simulink model "TST_AirHt_Ctl"  (R2016b)
settings: Solver=FixedStepDiscrete  StartTime=0.0  StopTime=simTime  FixedStep=sampleTime  RelTol=1e-3
values from neighbouring files (symbols this model uses):
  testCase = 1    [initTST_AirHt_Ctl_001.m]    (also in initTST_AirHt_Ctl_002.m = 2; initTST_AirHt_Ctl_003.m = 3; initTST_AirHt_Ctl_004.m = 4; initTST_AirHt_Ctl_005.m = 5)
libraries: simulink x53, UnitTest_Lib x26
(part 1 of 4)
settings Model: Creator=zhengjinyan  LastModifiedBy=zhengjinyan
settings DebuggingCC: SignalRangeChecking=error

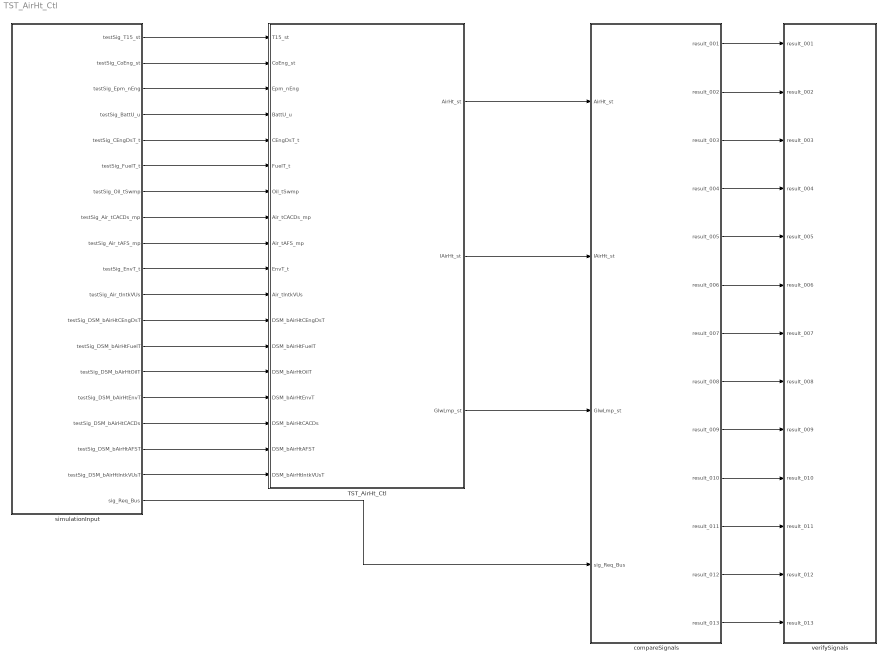
== system TST_AirHt_Ctl ==
  TST_AirHt_Ctl : Subsystem
  compareSignals : Subsystem
  simulationInput : Subsystem
  verifySignals : Subsystem
  wires:
  simulationInput/1(testSig_T15_st) -> TST_AirHt_Ctl/1(T15_st)
  simulationInput/2(testSig_CoEng_st) -> TST_AirHt_Ctl/2(CoEng_st)
  simulationInput/3(testSig_Epm_nEng) -> TST_AirHt_Ctl/3(Epm_nEng)
  simulationInput/4(testSig_BattU_u) -> TST_AirHt_Ctl/4(BattU_u)
  simulationInput/5(testSig_CEngDsT_t) -> TST_AirHt_Ctl/5(CEngDsT_t)
  simulationInput/6(testSig_FuelT_t) -> TST_AirHt_Ctl/6(FuelT_t)
  simulationInput/7(testSig_Oil_tSwmp) -> TST_AirHt_Ctl/7(Oil_tSwmp)
  simulationInput/8(testSig_Air_tCACDs_mp) -> TST_AirHt_Ctl/8(Air_tCACDs_mp)
  simulationInput/9(testSig_Air_tAFS_mp) -> TST_AirHt_Ctl/9(Air_tAFS_mp)
  simulationInput/10(testSig_EnvT_t) -> TST_AirHt_Ctl/10(EnvT_t)
  simulationInput/11(testSig_Air_tIntkVUs) -> TST_AirHt_Ctl/11(Air_tIntkVUs)
  simulationInput/12(testSig_DSM_bAirHtCEngDsT) -> TST_AirHt_Ctl/12(DSM_bAirHtCEngDsT)
  simulationInput/13(testSig_DSM_bAirHtFuelT) -> TST_AirHt_Ctl/13(DSM_bAirHtFuelT)
  simulationInput/14(testSig_DSM_bAirHtOilT) -> TST_AirHt_Ctl/14(DSM_bAirHtOilT)
  simulationInput/15(testSig_DSM_bAirHtEnvT) -> TST_AirHt_Ctl/15(DSM_bAirHtEnvT)
  simulationInput/16(testSig_DSM_bAirHtCACDs) -> TST_AirHt_Ctl/16(DSM_bAirHtCACDs)
  simulationInput/17(testSig_DSM_bAirHtAFST) -> TST_AirHt_Ctl/17(DSM_bAirHtAFST)
  simulationInput/18(testSig_DSM_bAirHtIntkVUsT) -> TST_AirHt_Ctl/18(DSM_bAirHtIntkVUsT)
  TST_AirHt_Ctl/1(AirHt_st) -> compareSignals/1(AirHt_st)
  TST_AirHt_Ctl/2(IAirHt_st) -> compareSignals/2(IAirHt_st)
  TST_AirHt_Ctl/3(GlwLmp_st) -> compareSignals/3(GlwLmp_st)
  simulationInput/19(sig_Req_Bus) -> compareSignals/4(sig_Req_Bus)
  compareSignals/1(result_001) -> verifySignals/1(result_001)
  compareSignals/2(result_002) -> verifySignals/2(result_002)
  compareSignals/3(result_003) -> verifySignals/3(result_003)
  compareSignals/4(result_004) -> verifySignals/4(result_004)
  compareSignals/5(result_005) -> verifySignals/5(result_005)
  compareSignals/6(result_006) -> verifySignals/6(result_006)
  compareSignals/7(result_007) -> verifySignals/7(result_007)
  compareSignals/8(result_008) -> verifySignals/8(result_008)
  compareSignals/9(result_009) -> verifySignals/9(result_009)
  compareSignals/10(result_010) -> verifySignals/10(result_010)
  compareSignals/11(result_011) -> verifySignals/11(result_011)
  compareSignals/12(result_012) -> verifySignals/12(result_012)
  compareSignals/13(result_013) -> verifySignals/13(result_013)

== system TST_AirHt_Ctl/TST_AirHt_Ctl ==
  T15_st : Inport
  CoEng_st : Inport  Port=2
  Epm_nEng : Inport  Port=3
  BattU_u : Inport  Port=4
  CEngDsT_t : Inport  Port=5
  FuelT_t : Inport  Port=6
  Oil_tSwmp : Inport  Port=7
  Air_tCACDs_mp : Inport  Port=8
  Air_tAFS_mp : Inport  Port=9
  EnvT_t : Inport  Port=10
  Air_tIntkVUs : Inport  Port=11
  DSM_bAirHtCEngDsT : Inport  Port=12
  DSM_bAirHtFuelT : Inport  Port=13
  DSM_bAirHtOilT : Inport  Port=14
  DSM_bAirHtEnvT : Inport  Port=15
  DSM_bAirHtCACDs : Inport  Port=16
  DSM_bAirHtAFST : Inport  Port=17
  DSM_bAirHtIntkVUsT : Inport  Port=18
  AirHt_Ctl : ModelReference  ModelNameDialog=AirHt_Ctl  SimulationMode=Normal  ModelReferenceVersion=1.145  TriggerPortName=function  TriggerPortTriggerType=function-call  TriggerPortStatesWhenEnabling=held
  Function_Call : simulink/Ports & Subsystems/Function-Call Generator  sample_time=sampleTime  numberOfIterations=1
  AirHt_st : Outport
  IAirHt_st : Outport  Port=2
  GlwLmp_st : Outport  Port=3
  wires:
  Function_Call/1 -> AirHt_Ctl/Trigger
  T15_st/1 -> AirHt_Ctl/1
  CoEng_st/1 -> AirHt_Ctl/2
  Epm_nEng/1 -> AirHt_Ctl/3
  BattU_u/1 -> AirHt_Ctl/4
  CEngDsT_t/1 -> AirHt_Ctl/5
  FuelT_t/1 -> AirHt_Ctl/6
  Oil_tSwmp/1 -> AirHt_Ctl/7
  Air_tCACDs_mp/1 -> AirHt_Ctl/8
  Air_tAFS_mp/1 -> AirHt_Ctl/9
  EnvT_t/1 -> AirHt_Ctl/10
  Air_tIntkVUs/1 -> AirHt_Ctl/11
  DSM_bAirHtCEngDsT/1 -> AirHt_Ctl/12
  DSM_bAirHtFuelT/1 -> AirHt_Ctl/13
  DSM_bAirHtOilT/1 -> AirHt_Ctl/14
  DSM_bAirHtEnvT/1 -> AirHt_Ctl/15
  DSM_bAirHtCACDs/1 -> AirHt_Ctl/16
  DSM_bAirHtAFST/1 -> AirHt_Ctl/17
  DSM_bAirHtIntkVUsT/1 -> AirHt_Ctl/18
  AirHt_Ctl/1 -> AirHt_st/1
  AirHt_Ctl/2 -> IAirHt_st/1
  AirHt_Ctl/3 -> GlwLmp_st/1

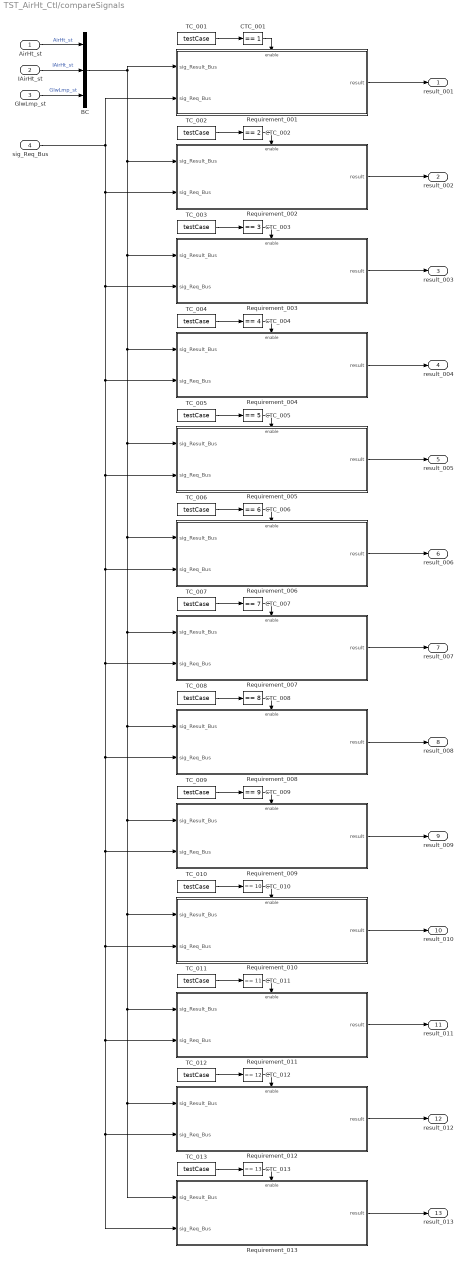
== system TST_AirHt_Ctl/compareSignals ==
  AirHt_st : Inport
  IAirHt_st : Inport  Port=2
  GlwLmp_st : Inport  Port=3
  sig_Req_Bus : Inport  Port=4
  BC : BusCreator  Inputs=3
  CTC_001 : simulink/Logic and Bit Operations/Compare To Constant  relop===  const=1  OutDataTypeStr=boolean
  CTC_002 : simulink/Logic and Bit Operations/Compare To Constant  relop===  const=2  OutDataTypeStr=boolean
  CTC_003 : simulink/Logic and Bit Operations/Compare To Constant  relop===  const=3  OutDataTypeStr=boolean
  CTC_004 : simulink/Logic and Bit Operations/Compare To Constant  relop===  const=4  OutDataTypeStr=boolean
  CTC_005 : simulink/Logic and Bit Operations/Compare To Constant  relop===  const=5  OutDataTypeStr=boolean
  CTC_006 : simulink/Logic and Bit Operations/Compare To Constant  relop===  const=6  OutDataTypeStr=boolean
  CTC_007 : simulink/Logic and Bit Operations/Compare To Constant  relop===  const=7  OutDataTypeStr=boolean
  CTC_008 : simulink/Logic and Bit Operations/Compare To Constant  relop===  const=8  OutDataTypeStr=boolean
  CTC_009 : simulink/Logic and Bit Operations/Compare To Constant  relop===  const=9  OutDataTypeStr=boolean
  CTC_010 : simulink/Logic and Bit Operations/Compare To Constant  relop===  const=10  OutDataTypeStr=boolean
  CTC_011 : simulink/Logic and Bit Operations/Compare To Constant  relop===  const=11  OutDataTypeStr=boolean
  CTC_012 : simulink/Logic and Bit Operations/Compare To Constant  relop===  const=12  OutDataTypeStr=boolean
  CTC_013 : simulink/Logic and Bit Operations/Compare To Constant  relop===  const=13  OutDataTypeStr=boolean
  Requirement_001 : Subsystem
  Requirement_002 : Subsystem
  Requirement_003 : Subsystem
  Requirement_004 : Subsystem
  Requirement_005 : Subsystem
  Requirement_006 : Subsystem
  Requirement_007 : Subsystem
  Requirement_008 : Subsystem
  Requirement_009 : Subsystem
  Requirement_010 : Subsystem
  Requirement_011 : Subsystem
  Requirement_012 : Subsystem
  Requirement_013 : Subsystem
  TC_001 : Constant  Value=testCase
  TC_002 : Constant  Value=testCase
  TC_003 : Constant  Value=testCase
  TC_004 : Constant  Value=testCase
  TC_005 : Constant  Value=testCase
  TC_006 : Constant  Value=testCase
  TC_007 : Constant  Value=testCase
  TC_008 : Constant  Value=testCase
  TC_009 : Constant  Value=testCase
  TC_010 : Constant  Value=testCase
  TC_011 : Constant  Value=testCase
  TC_012 : Constant  Value=testCase
  TC_013 : Constant  Value=testCase
  result_001 : Outport
  result_002 : Outport  Port=2
  result_003 : Outport  Port=3
  result_004 : Outport  Port=4
  result_005 : Outport  Port=5
  result_006 : Outport  Port=6
  result_007 : Outport  Port=7
  result_008 : Outport  Port=8
  result_009 : Outport  Port=9
  result_010 : Outport  Port=10
  result_011 : Outport  Port=11
  result_012 : Outport  Port=12
  result_013 : Outport  Port=13
  wires:
  AirHt_st/1 -> BC/1  "AirHt_st"
  IAirHt_st/1 -> BC/2  "IAirHt_st"
  GlwLmp_st/1 -> BC/3  "GlwLmp_st"
  TC_001/1 -> CTC_001/1
  CTC_001/1 -> Requirement_001/Enable
  sig_Req_Bus/1 -> Requirement_012/2(sig_Req_Bus), Requirement_013/2(sig_Req_Bus), Requirement_011/2(sig_Req_Bus), Requirement_010/2(sig_Req_Bus), Requirement_009/2(sig_Req_Bus), Requirement_008/2(sig_Req_Bus), Requirement_007/2(sig_Req_Bus), Requirement_006/2(sig_Req_Bus), Requirement_005/2(sig_Req_Bus), Requirement_004/2(sig_Req_Bus), Requirement_003/2(sig_Req_Bus), Requirement_002/2(sig_Req_Bus), Requirement_001/2(sig_Req_Bus)
  BC/1 -> Requirement_012/1(sig_Result_Bus), Requirement_013/1(sig_Result_Bus), Requirement_011/1(sig_Result_Bus), Requirement_010/1(sig_Result_Bus), Requirement_009/1(sig_Result_Bus), Requirement_008/1(sig_Result_Bus), Requirement_007/1(sig_Result_Bus), Requirement_006/1(sig_Result_Bus), Requirement_005/1(sig_Result_Bus), Requirement_004/1(sig_Result_Bus), Requirement_003/1(sig_Result_Bus), Requirement_002/1(sig_Result_Bus), Requirement_001/1(sig_Result_Bus)
  Requirement_001/1(result) -> result_001/1
  TC_002/1 -> CTC_002/1
  CTC_002/1 -> Requirement_002/Enable
  Requirement_002/1(result) -> result_002/1
  TC_003/1 -> CTC_003/1
  CTC_003/1 -> Requirement_003/Enable
  Requirement_003/1(result) -> result_003/1
  TC_004/1 -> CTC_004/1
  CTC_004/1 -> Requirement_004/Enable
  Requirement_004/1(result) -> result_004/1
  TC_005/1 -> CTC_005/1
  CTC_005/1 -> Requirement_005/Enable
  Requirement_005/1(result) -> result_005/1
  TC_006/1 -> CTC_006/1
  CTC_006/1 -> Requirement_006/Enable
  Requirement_006/1(result) -> result_006/1
  TC_007/1 -> CTC_007/1
  CTC_007/1 -> Requirement_007/Enable
  Requirement_007/1(result) -> result_007/1
  TC_008/1 -> CTC_008/1
  CTC_008/1 -> Requirement_008/Enable
  Requirement_008/1(result) -> result_008/1
  TC_009/1 -> CTC_009/1
  CTC_009/1 -> Requirement_009/Enable
  Requirement_009/1(result) -> result_009/1
  TC_010/1 -> CTC_010/1
  CTC_010/1 -> Requirement_010/Enable
  Requirement_010/1(result) -> result_010/1
  TC_011/1 -> CTC_011/1
  CTC_011/1 -> Requirement_011/Enable
  Requirement_011/1(result) -> result_011/1
  TC_012/1 -> CTC_012/1
  CTC_012/1 -> Requirement_012/Enable
  Requirement_012/1(result) -> result_012/1
  TC_013/1 -> CTC_013/1
  CTC_013/1 -> Requirement_013/Enable
  Requirement_013/1(result) -> result_013/1

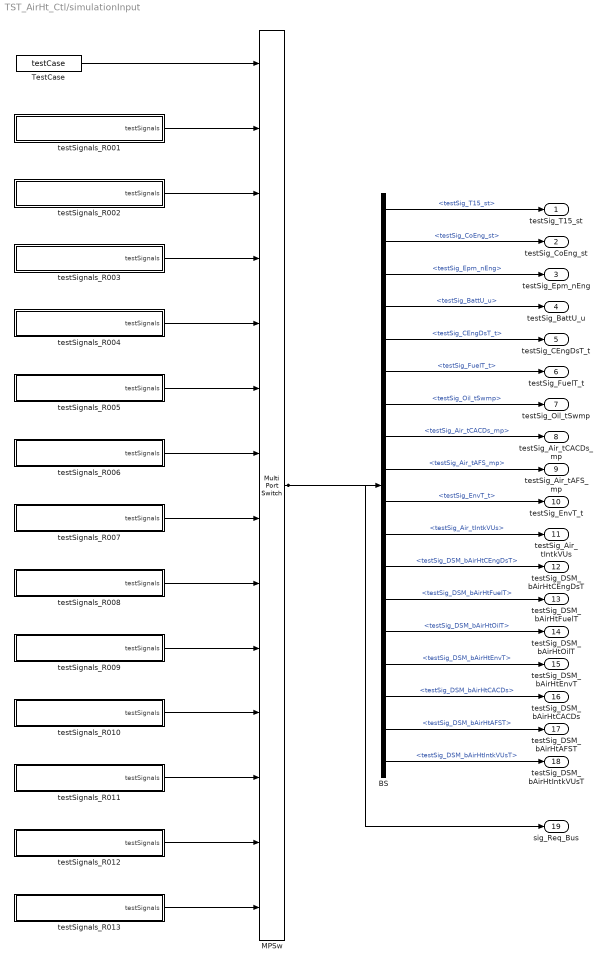
== system TST_AirHt_Ctl/simulationInput ==
  BS : BusSelector  OutputSignals=testSig_T15_st,testSig_CoEng_st,testSig_Epm_nEng,testSig_BattU_u,testSig_CEngDsT_t,testSig_FuelT_t,testSig_Oil_tSwmp,testSig_Air_tCACDs_mp,testSig_Air_tAFS_mp,testSig_EnvT_t,testSig_Air_tIntkVUs,testSig_DSM_bAirHtCEngDsT,testSig_DSM_bAirHtFuelT,testSig_DSM_bAirHtOilT,testSig_DSM_bAirHtEnvT,testSig_DSM_bAirHtCACDs,testSig_DSM_bAirHtAFST,testSig_DSM_bAirHtIntkVUsT
  MPSw : MultiPortSwitch  Inputs=13  SaturateOnIntegerOverflow=on  InputSameDT=on
  TestCase : Constant  Value=testCase
  testSignals_R001 : Subsystem
  testSignals_R002 : Subsystem
  testSignals_R003 : Subsystem
  testSignals_R004 : Subsystem
  testSignals_R005 : Subsystem
  testSignals_R006 : Subsystem
  testSignals_R007 : Subsystem
  testSignals_R008 : Subsystem
  testSignals_R009 : Subsystem
  testSignals_R010 : Subsystem
  testSignals_R011 : Subsystem
  testSignals_R012 : Subsystem
  testSignals_R013 : Subsystem
  testSig_T15_st : Outport
  testSig_CoEng_st : Outport  Port=2
  testSig_Epm_nEng : Outport  Port=3
  testSig_BattU_u : Outport  Port=4
  testSig_CEngDsT_t : Outport  Port=5
  testSig_FuelT_t : Outport  Port=6
  testSig_Oil_tSwmp : Outport  Port=7
  testSig_Air_tCACDs_mp : Outport  Port=8
  testSig_Air_tAFS_mp : Outport  Port=9
  testSig_EnvT_t : Outport  Port=10
  testSig_Air_tIntkVUs : Outport  Port=11
  testSig_DSM_bAirHtCEngDsT : Outport  Port=12
  testSig_DSM_bAirHtFuelT : Outport  Port=13
  testSig_DSM_bAirHtOilT : Outport  Port=14
  testSig_DSM_bAirHtEnvT : Outport  Port=15
  testSig_DSM_bAirHtCACDs : Outport  Port=16
  testSig_DSM_bAirHtAFST : Outport  Port=17
  testSig_DSM_bAirHtIntkVUsT : Outport  Port=18
  sig_Req_Bus : Outport  Port=19
  wires:
  BS/1 -> testSig_T15_st/1  "<testSig_T15_st>"
  BS/2 -> testSig_CoEng_st/1  "<testSig_CoEng_st>"
  BS/3 -> testSig_Epm_nEng/1  "<testSig_Epm_nEng>"
  BS/4 -> testSig_BattU_u/1  "<testSig_BattU_u>"
  BS/5 -> testSig_CEngDsT_t/1  "<testSig_CEngDsT_t>"
  BS/6 -> testSig_FuelT_t/1  "<testSig_FuelT_t>"
  BS/7 -> testSig_Oil_tSwmp/1  "<testSig_Oil_tSwmp>"
  BS/8 -> testSig_Air_tCACDs_mp/1  "<testSig_Air_tCACDs_mp>"
  BS/9 -> testSig_Air_tAFS_mp/1  "<testSig_Air_tAFS_mp>"
  BS/10 -> testSig_EnvT_t/1  "<testSig_EnvT_t>"
  BS/11 -> testSig_Air_tIntkVUs/1  "<testSig_Air_tIntkVUs>"
  BS/12 -> testSig_DSM_bAirHtCEngDsT/1  "<testSig_DSM_bAirHtCEngDsT>"
  BS/13 -> testSig_DSM_bAirHtFuelT/1  "<testSig_DSM_bAirHtFuelT>"
  BS/14 -> testSig_DSM_bAirHtOilT/1  "<testSig_DSM_bAirHtOilT>"
  BS/15 -> testSig_DSM_bAirHtEnvT/1  "<testSig_DSM_bAirHtEnvT>"
  BS/16 -> testSig_DSM_bAirHtCACDs/1  "<testSig_DSM_bAirHtCACDs>"
  BS/17 -> testSig_DSM_bAirHtAFST/1  "<testSig_DSM_bAirHtAFST>"
  BS/18 -> testSig_DSM_bAirHtIntkVUsT/1  "<testSig_DSM_bAirHtIntkVUsT>"
  MPSw/1 -> BS/1, sig_Req_Bus/1
  TestCase/1 -> MPSw/1
  testSignals_R001/1(testSignals) -> MPSw/2
  testSignals_R002/1(testSignals) -> MPSw/3
  testSignals_R003/1(testSignals) -> MPSw/4
  testSignals_R004/1(testSignals) -> MPSw/5
  testSignals_R005/1(testSignals) -> MPSw/6
  testSignals_R006/1(testSignals) -> MPSw/7
  testSignals_R007/1(testSignals) -> MPSw/8
  testSignals_R008/1(testSignals) -> MPSw/9
  testSignals_R009/1(testSignals) -> MPSw/10
  testSignals_R010/1(testSignals) -> MPSw/11
  testSignals_R011/1(testSignals) -> MPSw/12
  testSignals_R012/1(testSignals) -> MPSw/13
  testSignals_R013/1(testSignals) -> MPSw/14

== system TST_AirHt_Ctl/verifySignals ==
  result_001 : Inport
  result_002 : Inport  Port=2
  result_003 : Inport  Port=3
  result_004 : Inport  Port=4
  result_005 : Inport  Port=5
  result_006 : Inport  Port=6
  result_007 : Inport  Port=7
  result_008 : Inport  Port=8
  result_009 : Inport  Port=9
  result_010 : Inport  Port=10
  result_011 : Inport  Port=11
  result_012 : Inport  Port=12
  result_013 : Inport  Port=13
  Assertion_001 : Assertion  Enabled=off
  Assertion_002 : Assertion  Enabled=off
  Assertion_003 : Assertion  Enabled=off
  Assertion_004 : Assertion  Enabled=off
  Assertion_005 : Assertion  Enabled=off
  Assertion_006 : Assertion  Enabled=off
  Assertion_007 : Assertion  Enabled=off
  Assertion_008 : Assertion  Enabled=off
  Assertion_009 : Assertion  Enabled=off
  Assertion_010 : Assertion  Enabled=off
  Assertion_011 : Assertion  Enabled=off
  Assertion_012 : Assertion  Enabled=off
  Assertion_013 : Assertion  Enabled=off
  wires:
  result_001/1 -> Assertion_001/1
  result_002/1 -> Assertion_002/1
  result_003/1 -> Assertion_003/1
  result_004/1 -> Assertion_004/1
  result_005/1 -> Assertion_005/1
  result_006/1 -> Assertion_006/1
  result_007/1 -> Assertion_007/1
  result_008/1 -> Assertion_008/1
  result_009/1 -> Assertion_009/1
  result_010/1 -> Assertion_010/1
  result_011/1 -> Assertion_011/1
  result_012/1 -> Assertion_012/1
  result_013/1 -> Assertion_013/1

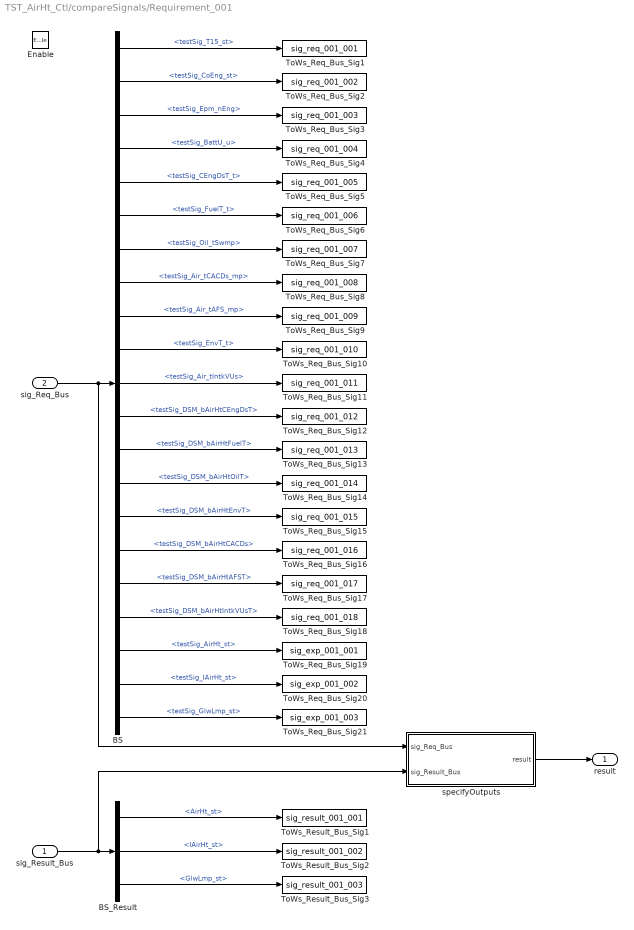
== system TST_AirHt_Ctl/compareSignals/Requirement_001 ==
  sig_Result_Bus : Inport
  sig_Req_Bus : Inport  Port=2
  Enable : EnablePort
  BS : BusSelector  OutputSignals=testSig_T15_st,testSig_CoEng_st,testSig_Epm_nEng,testSig_BattU_u,testSig_CEngDsT_t,testSig_FuelT_t,testSig_Oil_tSwmp,testSig_Air_tCACDs_mp,testSig_Air_tAFS_mp,testSig_EnvT_t,testSig_Air_tIntkVUs,testSig_DSM_bAirHtCEngDsT,testSig_DSM_bAirHtFuelT,testSig_DSM_bAirHtOilT,testSig_DSM_bAirHtEnvT,testSig_DSM_bAirHtCACDs,testSig_DSM_bAirHtAFST,testSig_DSM_bAirHtIntkVUsT,testSig_AirHt_st,testSig_IAirHt_st,testSig_GlwLmp_st
  BS_Result : BusSelector  OutputSignals=AirHt_st,IAirHt_st,GlwLmp_st
  ToWs_Req_Bus_Sig1 : ToWorkspace  VariableName=sig_req_001_001  SaveFormat=Structure With Time
  ToWs_Req_Bus_Sig10 : ToWorkspace  VariableName=sig_req_001_010  SaveFormat=Structure With Time
  ToWs_Req_Bus_Sig11 : ToWorkspace  VariableName=sig_req_001_011  SaveFormat=Structure With Time
  ToWs_Req_Bus_Sig12 : ToWorkspace  VariableName=sig_req_001_012  SaveFormat=Structure With Time
  ToWs_Req_Bus_Sig13 : ToWorkspace  VariableName=sig_req_001_013  SaveFormat=Structure With Time
  ToWs_Req_Bus_Sig14 : ToWorkspace  VariableName=sig_req_001_014  SaveFormat=Structure With Time
  ToWs_Req_Bus_Sig15 : ToWorkspace  VariableName=sig_req_001_015  SaveFormat=Structure With Time
  ToWs_Req_Bus_Sig16 : ToWorkspace  VariableName=sig_req_001_016  SaveFormat=Structure With Time
  ToWs_Req_Bus_Sig17 : ToWorkspace  VariableName=sig_req_001_017  SaveFormat=Structure With Time
  ToWs_Req_Bus_Sig18 : ToWorkspace  VariableName=sig_req_001_018  SaveFormat=Structure With Time
  ToWs_Req_Bus_Sig19 : ToWorkspace  VariableName=sig_exp_001_001  SaveFormat=Structure With Time
  ToWs_Req_Bus_Sig2 : ToWorkspace  VariableName=sig_req_001_002  SaveFormat=Structure With Time
  ToWs_Req_Bus_Sig20 : ToWorkspace  VariableName=sig_exp_001_002  SaveFormat=Structure With Time
  ToWs_Req_Bus_Sig21 : ToWorkspace  VariableName=sig_exp_001_003  SaveFormat=Structure With Time
  ToWs_Req_Bus_Sig3 : ToWorkspace  VariableName=sig_req_001_003  SaveFormat=Structure With Time
  ToWs_Req_Bus_Sig4 : ToWorkspace  VariableName=sig_req_001_004  SaveFormat=Structure With Time
  ToWs_Req_Bus_Sig5 : ToWorkspace  VariableName=sig_req_001_005  SaveFormat=Structure With Time
  ToWs_Req_Bus_Sig6 : ToWorkspace  VariableName=sig_req_001_006  SaveFormat=Structure With Time
  ToWs_Req_Bus_Sig7 : ToWorkspace  VariableName=sig_req_001_007  SaveFormat=Structure With Time
  ToWs_Req_Bus_Sig8 : ToWorkspace  VariableName=sig_req_001_008  SaveFormat=Structure With Time
  ToWs_Req_Bus_Sig9 : ToWorkspace  VariableName=sig_req_001_009  SaveFormat=Structure With Time
  ToWs_Result_Bus_Sig1 : ToWorkspace  VariableName=sig_result_001_001  SaveFormat=Structure With Time
  ToWs_Result_Bus_Sig2 : ToWorkspace  VariableName=sig_result_001_002  SaveFormat=Structure With Time
  ToWs_Result_Bus_Sig3 : ToWorkspace  VariableName=sig_result_001_003  SaveFormat=Structure With Time
  specifyOutputs : Subsystem
  result : Outport
  wires:
  sig_Req_Bus/1 -> BS/1, specifyOutputs/1(sig_Req_Bus)
  BS/1 -> ToWs_Req_Bus_Sig1/1  "<testSig_T15_st>"
  BS/2 -> ToWs_Req_Bus_Sig2/1  "<testSig_CoEng_st>"
  BS/3 -> ToWs_Req_Bus_Sig3/1  "<testSig_Epm_nEng>"
  BS/4 -> ToWs_Req_Bus_Sig4/1  "<testSig_BattU_u>"
  BS/5 -> ToWs_Req_Bus_Sig5/1  "<testSig_CEngDsT_t>"
  BS/6 -> ToWs_Req_Bus_Sig6/1  "<testSig_FuelT_t>"
  BS/7 -> ToWs_Req_Bus_Sig7/1  "<testSig_Oil_tSwmp>"
  BS/8 -> ToWs_Req_Bus_Sig8/1  "<testSig_Air_tCACDs_mp>"
  BS/9 -> ToWs_Req_Bus_Sig9/1  "<testSig_Air_tAFS_mp>"
  BS/10 -> ToWs_Req_Bus_Sig10/1  "<testSig_EnvT_t>"
  BS/11 -> ToWs_Req_Bus_Sig11/1  "<testSig_Air_tIntkVUs>"
  BS/12 -> ToWs_Req_Bus_Sig12/1  "<testSig_DSM_bAirHtCEngDsT>"
  BS/13 -> ToWs_Req_Bus_Sig13/1  "<testSig_DSM_bAirHtFuelT>"
  BS/14 -> ToWs_Req_Bus_Sig14/1  "<testSig_DSM_bAirHtOilT>"
  BS/15 -> ToWs_Req_Bus_Sig15/1  "<testSig_DSM_bAirHtEnvT>"
  BS/16 -> ToWs_Req_Bus_Sig16/1  "<testSig_DSM_bAirHtCACDs>"
  BS/17 -> ToWs_Req_Bus_Sig17/1  "<testSig_DSM_bAirHtAFST>"
  BS/18 -> ToWs_Req_Bus_Sig18/1  "<testSig_DSM_bAirHtIntkVUsT>"
  BS/19 -> ToWs_Req_Bus_Sig19/1  "<testSig_AirHt_st>"
  BS/20 -> ToWs_Req_Bus_Sig20/1  "<testSig_IAirHt_st>"
  BS/21 -> ToWs_Req_Bus_Sig21/1  "<testSig_GlwLmp_st>"
  sig_Result_Bus/1 -> BS_Result/1, specifyOutputs/2(sig_Result_Bus)
  BS_Result/1 -> ToWs_Result_Bus_Sig1/1  "<AirHt_st>"
  BS_Result/2 -> ToWs_Result_Bus_Sig2/1  "<IAirHt_st>"
  BS_Result/3 -> ToWs_Result_Bus_Sig3/1  "<GlwLmp_st>"
  specifyOutputs/1(result) -> result/1

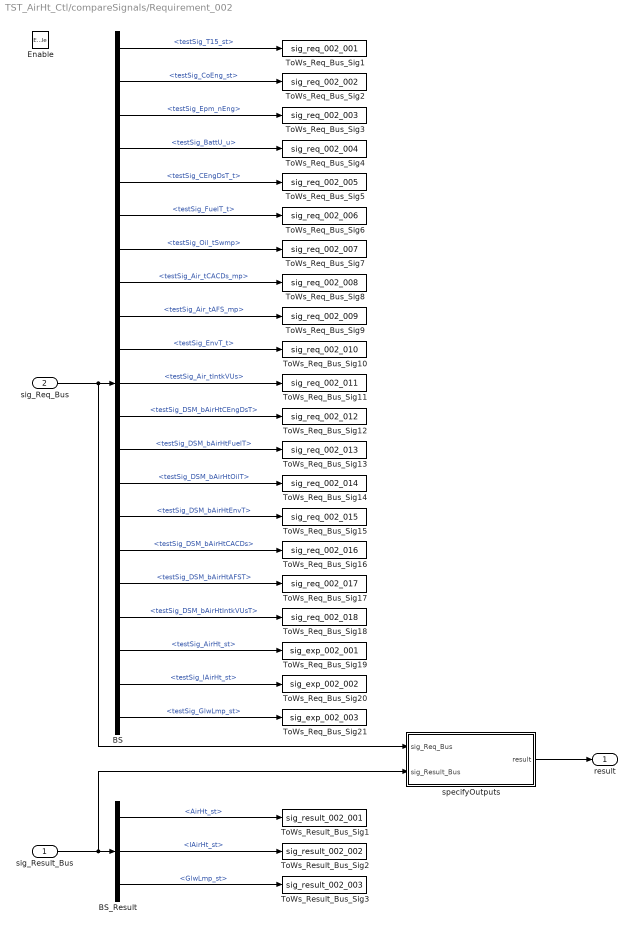
== system TST_AirHt_Ctl/compareSignals/Requirement_002 ==
  sig_Result_Bus : Inport
  sig_Req_Bus : Inport  Port=2
  Enable : EnablePort
  BS : BusSelector  OutputSignals=testSig_T15_st,testSig_CoEng_st,testSig_Epm_nEng,testSig_BattU_u,testSig_CEngDsT_t,testSig_FuelT_t,testSig_Oil_tSwmp,testSig_Air_tCACDs_mp,testSig_Air_tAFS_mp,testSig_EnvT_t,testSig_Air_tIntkVUs,testSig_DSM_bAirHtCEngDsT,testSig_DSM_bAirHtFuelT,testSig_DSM_bAirHtOilT,testSig_DSM_bAirHtEnvT,testSig_DSM_bAirHtCACDs,testSig_DSM_bAirHtAFST,testSig_DSM_bAirHtIntkVUsT,testSig_AirHt_st,testSig_IAirHt_st,testSig_GlwLmp_st
  BS_Result : BusSelector  OutputSignals=AirHt_st,IAirHt_st,GlwLmp_st
  ToWs_Req_Bus_Sig1 : ToWorkspace  VariableName=sig_req_002_001  SaveFormat=Structure With Time
  ToWs_Req_Bus_Sig10 : ToWorkspace  VariableName=sig_req_002_010  SaveFormat=Structure With Time
  ToWs_Req_Bus_Sig11 : ToWorkspace  VariableName=sig_req_002_011  SaveFormat=Structure With Time
  ToWs_Req_Bus_Sig12 : ToWorkspace  VariableName=sig_req_002_012  SaveFormat=Structure With Time
  ToWs_Req_Bus_Sig13 : ToWorkspace  VariableName=sig_req_002_013  SaveFormat=Structure With Time
  ToWs_Req_Bus_Sig14 : ToWorkspace  VariableName=sig_req_002_014  SaveFormat=Structure With Time
  ToWs_Req_Bus_Sig15 : ToWorkspace  VariableName=sig_req_002_015  SaveFormat=Structure With Time
  ToWs_Req_Bus_Sig16 : ToWorkspace  VariableName=sig_req_002_016  SaveFormat=Structure With Time
  ToWs_Req_Bus_Sig17 : ToWorkspace  VariableName=sig_req_002_017  SaveFormat=Structure With Time
  ToWs_Req_Bus_Sig18 : ToWorkspace  VariableName=sig_req_002_018  SaveFormat=Structure With Time
  ToWs_Req_Bus_Sig19 : ToWorkspace  VariableName=sig_exp_002_001  SaveFormat=Structure With Time
  ToWs_Req_Bus_Sig2 : ToWorkspace  VariableName=sig_req_002_002  SaveFormat=Structure With Time
  ToWs_Req_Bus_Sig20 : ToWorkspace  VariableName=sig_exp_002_002  SaveFormat=Structure With Time
  ToWs_Req_Bus_Sig21 : ToWorkspace  VariableName=sig_exp_002_003  SaveFormat=Structure With Time
  ToWs_Req_Bus_Sig3 : ToWorkspace  VariableName=sig_req_002_003  SaveFormat=Structure With Time
  ToWs_Req_Bus_Sig4 : ToWorkspace  VariableName=sig_req_002_004  SaveFormat=Structure With Time
  ToWs_Req_Bus_Sig5 : ToWorkspace  VariableName=sig_req_002_005  SaveFormat=Structure With Time
  ToWs_Req_Bus_Sig6 : ToWorkspace  VariableName=sig_req_002_006  SaveFormat=Structure With Time
  ToWs_Req_Bus_Sig7 : ToWorkspace  VariableName=sig_req_002_007  SaveFormat=Structure With Time
  ToWs_Req_Bus_Sig8 : ToWorkspace  VariableName=sig_req_002_008  SaveFormat=Structure With Time
  ToWs_Req_Bus_Sig9 : ToWorkspace  VariableName=sig_req_002_009  SaveFormat=Structure With Time
  ToWs_Result_Bus_Sig1 : ToWorkspace  VariableName=sig_result_002_001  SaveFormat=Structure With Time
  ToWs_Result_Bus_Sig2 : ToWorkspace  VariableName=sig_result_002_002  SaveFormat=Structure With Time
  ToWs_Result_Bus_Sig3 : ToWorkspace  VariableName=sig_result_002_003  SaveFormat=Structure With Time
  specifyOutputs : Subsystem
  result : Outport
  wires:
  sig_Req_Bus/1 -> BS/1, specifyOutputs/1(sig_Req_Bus)
  BS/1 -> ToWs_Req_Bus_Sig1/1  "<testSig_T15_st>"
  BS/2 -> ToWs_Req_Bus_Sig2/1  "<testSig_CoEng_st>"
  BS/3 -> ToWs_Req_Bus_Sig3/1  "<testSig_Epm_nEng>"
  BS/4 -> ToWs_Req_Bus_Sig4/1  "<testSig_BattU_u>"
  BS/5 -> ToWs_Req_Bus_Sig5/1  "<testSig_CEngDsT_t>"
  BS/6 -> ToWs_Req_Bus_Sig6/1  "<testSig_FuelT_t>"
  BS/7 -> ToWs_Req_Bus_Sig7/1  "<testSig_Oil_tSwmp>"
  BS/8 -> ToWs_Req_Bus_Sig8/1  "<testSig_Air_tCACDs_mp>"
  BS/9 -> ToWs_Req_Bus_Sig9/1  "<testSig_Air_tAFS_mp>"
  BS/10 -> ToWs_Req_Bus_Sig10/1  "<testSig_EnvT_t>"
  BS/11 -> ToWs_Req_Bus_Sig11/1  "<testSig_Air_tIntkVUs>"
  BS/12 -> ToWs_Req_Bus_Sig12/1  "<testSig_DSM_bAirHtCEngDsT>"
  BS/13 -> ToWs_Req_Bus_Sig13/1  "<testSig_DSM_bAirHtFuelT>"
  BS/14 -> ToWs_Req_Bus_Sig14/1  "<testSig_DSM_bAirHtOilT>"
  BS/15 -> ToWs_Req_Bus_Sig15/1  "<testSig_DSM_bAirHtEnvT>"
  BS/16 -> ToWs_Req_Bus_Sig16/1  "<testSig_DSM_bAirHtCACDs>"
  BS/17 -> ToWs_Req_Bus_Sig17/1  "<testSig_DSM_bAirHtAFST>"
  BS/18 -> ToWs_Req_Bus_Sig18/1  "<testSig_DSM_bAirHtIntkVUsT>"
  BS/19 -> ToWs_Req_Bus_Sig19/1  "<testSig_AirHt_st>"
  BS/20 -> ToWs_Req_Bus_Sig20/1  "<testSig_IAirHt_st>"
  BS/21 -> ToWs_Req_Bus_Sig21/1  "<testSig_GlwLmp_st>"
  sig_Result_Bus/1 -> BS_Result/1, specifyOutputs/2(sig_Result_Bus)
  BS_Result/1 -> ToWs_Result_Bus_Sig1/1  "<AirHt_st>"
  BS_Result/2 -> ToWs_Result_Bus_Sig2/1  "<IAirHt_st>"
  BS_Result/3 -> ToWs_Result_Bus_Sig3/1  "<GlwLmp_st>"
  specifyOutputs/1(result) -> result/1

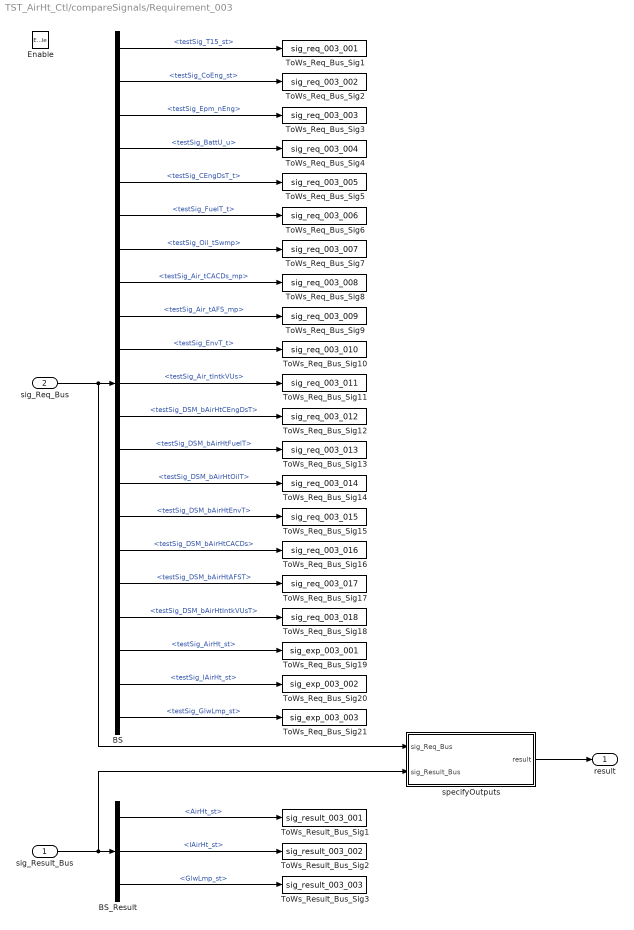
== system TST_AirHt_Ctl/compareSignals/Requirement_003 ==
  sig_Result_Bus : Inport
  sig_Req_Bus : Inport  Port=2
  Enable : EnablePort
  BS : BusSelector  OutputSignals=testSig_T15_st,testSig_CoEng_st,testSig_Epm_nEng,testSig_BattU_u,testSig_CEngDsT_t,testSig_FuelT_t,testSig_Oil_tSwmp,testSig_Air_tCACDs_mp,testSig_Air_tAFS_mp,testSig_EnvT_t,testSig_Air_tIntkVUs,testSig_DSM_bAirHtCEngDsT,testSig_DSM_bAirHtFuelT,testSig_DSM_bAirHtOilT,testSig_DSM_bAirHtEnvT,testSig_DSM_bAirHtCACDs,testSig_DSM_bAirHtAFST,testSig_DSM_bAirHtIntkVUsT,testSig_AirHt_st,testSig_IAirHt_st,testSig_GlwLmp_st
  BS_Result : BusSelector  OutputSignals=AirHt_st,IAirHt_st,GlwLmp_st
  ToWs_Req_Bus_Sig1 : ToWorkspace  VariableName=sig_req_003_001  SaveFormat=Structure With Time
  ToWs_Req_Bus_Sig10 : ToWorkspace  VariableName=sig_req_003_010  SaveFormat=Structure With Time
  ToWs_Req_Bus_Sig11 : ToWorkspace  VariableName=sig_req_003_011  SaveFormat=Structure With Time
  ToWs_Req_Bus_Sig12 : ToWorkspace  VariableName=sig_req_003_012  SaveFormat=Structure With Time
  ToWs_Req_Bus_Sig13 : ToWorkspace  VariableName=sig_req_003_013  SaveFormat=Structure With Time
  ToWs_Req_Bus_Sig14 : ToWorkspace  VariableName=sig_req_003_014  SaveFormat=Structure With Time
  ToWs_Req_Bus_Sig15 : ToWorkspace  VariableName=sig_req_003_015  SaveFormat=Structure With Time
  ToWs_Req_Bus_Sig16 : ToWorkspace  VariableName=sig_req_003_016  SaveFormat=Structure With Time
  ToWs_Req_Bus_Sig17 : ToWorkspace  VariableName=sig_req_003_017  SaveFormat=Structure With Time
  ToWs_Req_Bus_Sig18 : ToWorkspace  VariableName=sig_req_003_018  SaveFormat=Structure With Time
  ToWs_Req_Bus_Sig19 : ToWorkspace  VariableName=sig_exp_003_001  SaveFormat=Structure With Time
  ToWs_Req_Bus_Sig2 : ToWorkspace  VariableName=sig_req_003_002  SaveFormat=Structure With Time
  ToWs_Req_Bus_Sig20 : ToWorkspace  VariableName=sig_exp_003_002  SaveFormat=Structure With Time
  ToWs_Req_Bus_Sig21 : ToWorkspace  VariableName=sig_exp_003_003  SaveFormat=Structure With Time
  ToWs_Req_Bus_Sig3 : ToWorkspace  VariableName=sig_req_003_003  SaveFormat=Structure With Time
  ToWs_Req_Bus_Sig4 : ToWorkspace  VariableName=sig_req_003_004  SaveFormat=Structure With Time
  ToWs_Req_Bus_Sig5 : ToWorkspace  VariableName=sig_req_003_005  SaveFormat=Structure With Time
  ToWs_Req_Bus_Sig6 : ToWorkspace  VariableName=sig_req_003_006  SaveFormat=Structure With Time
  ToWs_Req_Bus_Sig7 : ToWorkspace  VariableName=sig_req_003_007  SaveFormat=Structure With Time
  ToWs_Req_Bus_Sig8 : ToWorkspace  VariableName=sig_req_003_008  SaveFormat=Structure With Time
  ToWs_Req_Bus_Sig9 : ToWorkspace  VariableName=sig_req_003_009  SaveFormat=Structure With Time
  ToWs_Result_Bus_Sig1 : ToWorkspace  VariableName=sig_result_003_001  SaveFormat=Structure With Time
  ToWs_Result_Bus_Sig2 : ToWorkspace  VariableName=sig_result_003_002  SaveFormat=Structure With Time
  ToWs_Result_Bus_Sig3 : ToWorkspace  VariableName=sig_result_003_003  SaveFormat=Structure With Time
  specifyOutputs : Subsystem
  result : Outport
  wires:
  sig_Req_Bus/1 -> BS/1, specifyOutputs/1(sig_Req_Bus)
  BS/1 -> ToWs_Req_Bus_Sig1/1  "<testSig_T15_st>"
  BS/2 -> ToWs_Req_Bus_Sig2/1  "<testSig_CoEng_st>"
  BS/3 -> ToWs_Req_Bus_Sig3/1  "<testSig_Epm_nEng>"
  BS/4 -> ToWs_Req_Bus_Sig4/1  "<testSig_BattU_u>"
  BS/5 -> ToWs_Req_Bus_Sig5/1  "<testSig_CEngDsT_t>"
  BS/6 -> ToWs_Req_Bus_Sig6/1  "<testSig_FuelT_t>"
  BS/7 -> ToWs_Req_Bus_Sig7/1  "<testSig_Oil_tSwmp>"
  BS/8 -> ToWs_Req_Bus_Sig8/1  "<testSig_Air_tCACDs_mp>"
  BS/9 -> ToWs_Req_Bus_Sig9/1  "<testSig_Air_tAFS_mp>"
  BS/10 -> ToWs_Req_Bus_Sig10/1  "<testSig_EnvT_t>"
  BS/11 -> ToWs_Req_Bus_Sig11/1  "<testSig_Air_tIntkVUs>"
  BS/12 -> ToWs_Req_Bus_Sig12/1  "<testSig_DSM_bAirHtCEngDsT>"
  BS/13 -> ToWs_Req_Bus_Sig13/1  "<testSig_DSM_bAirHtFuelT>"
  BS/14 -> ToWs_Req_Bus_Sig14/1  "<testSig_DSM_bAirHtOilT>"
  BS/15 -> ToWs_Req_Bus_Sig15/1  "<testSig_DSM_bAirHtEnvT>"
  BS/16 -> ToWs_Req_Bus_Sig16/1  "<testSig_DSM_bAirHtCACDs>"
  BS/17 -> ToWs_Req_Bus_Sig17/1  "<testSig_DSM_bAirHtAFST>"
  BS/18 -> ToWs_Req_Bus_Sig18/1  "<testSig_DSM_bAirHtIntkVUsT>"
  BS/19 -> ToWs_Req_Bus_Sig19/1  "<testSig_AirHt_st>"
  BS/20 -> ToWs_Req_Bus_Sig20/1  "<testSig_IAirHt_st>"
  BS/21 -> ToWs_Req_Bus_Sig21/1  "<testSig_GlwLmp_st>"
  sig_Result_Bus/1 -> BS_Result/1, specifyOutputs/2(sig_Result_Bus)
  BS_Result/1 -> ToWs_Result_Bus_Sig1/1  "<AirHt_st>"
  BS_Result/2 -> ToWs_Result_Bus_Sig2/1  "<IAirHt_st>"
  BS_Result/3 -> ToWs_Result_Bus_Sig3/1  "<GlwLmp_st>"
  specifyOutputs/1(result) -> result/1

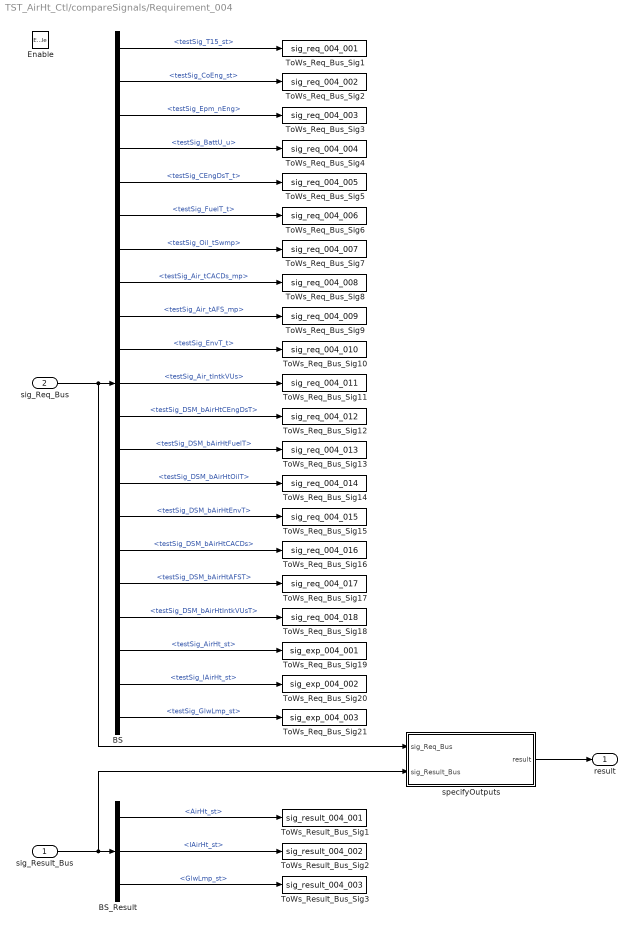
== system TST_AirHt_Ctl/compareSignals/Requirement_004 ==
  sig_Result_Bus : Inport
  sig_Req_Bus : Inport  Port=2
  Enable : EnablePort
  BS : BusSelector  OutputSignals=testSig_T15_st,testSig_CoEng_st,testSig_Epm_nEng,testSig_BattU_u,testSig_CEngDsT_t,testSig_FuelT_t,testSig_Oil_tSwmp,testSig_Air_tCACDs_mp,testSig_Air_tAFS_mp,testSig_EnvT_t,testSig_Air_tIntkVUs,testSig_DSM_bAirHtCEngDsT,testSig_DSM_bAirHtFuelT,testSig_DSM_bAirHtOilT,testSig_DSM_bAirHtEnvT,testSig_DSM_bAirHtCACDs,testSig_DSM_bAirHtAFST,testSig_DSM_bAirHtIntkVUsT,testSig_AirHt_st,testSig_IAirHt_st,testSig_GlwLmp_st
  BS_Result : BusSelector  OutputSignals=AirHt_st,IAirHt_st,GlwLmp_st
  ToWs_Req_Bus_Sig1 : ToWorkspace  VariableName=sig_req_004_001  SaveFormat=Structure With Time
  ToWs_Req_Bus_Sig10 : ToWorkspace  VariableName=sig_req_004_010  SaveFormat=Structure With Time
  ToWs_Req_Bus_Sig11 : ToWorkspace  VariableName=sig_req_004_011  SaveFormat=Structure With Time
  ToWs_Req_Bus_Sig12 : ToWorkspace  VariableName=sig_req_004_012  SaveFormat=Structure With Time
  ToWs_Req_Bus_Sig13 : ToWorkspace  VariableName=sig_req_004_013  SaveFormat=Structure With Time
  ToWs_Req_Bus_Sig14 : ToWorkspace  VariableName=sig_req_004_014  SaveFormat=Structure With Time
  ToWs_Req_Bus_Sig15 : ToWorkspace  VariableName=sig_req_004_015  SaveFormat=Structure With Time
  ToWs_Req_Bus_Sig16 : ToWorkspace  VariableName=sig_req_004_016  SaveFormat=Structure With Time
  ToWs_Req_Bus_Sig17 : ToWorkspace  VariableName=sig_req_004_017  SaveFormat=Structure With Time
  ToWs_Req_Bus_Sig18 : ToWorkspace  VariableName=sig_req_004_018  SaveFormat=Structure With Time
  ToWs_Req_Bus_Sig19 : ToWorkspace  VariableName=sig_exp_004_001  SaveFormat=Structure With Time
  ToWs_Req_Bus_Sig2 : ToWorkspace  VariableName=sig_req_004_002  SaveFormat=Structure With Time
  ToWs_Req_Bus_Sig20 : ToWorkspace  VariableName=sig_exp_004_002  SaveFormat=Structure With Time
  ToWs_Req_Bus_Sig21 : ToWorkspace  VariableName=sig_exp_004_003  SaveFormat=Structure With Time
  ToWs_Req_Bus_Sig3 : ToWorkspace  VariableName=sig_req_004_003  SaveFormat=Structure With Time
  ToWs_Req_Bus_Sig4 : ToWorkspace  VariableName=sig_req_004_004  SaveFormat=Structure With Time
  ToWs_Req_Bus_Sig5 : ToWorkspace  VariableName=sig_req_004_005  SaveFormat=Structure With Time
  ToWs_Req_Bus_Sig6 : ToWorkspace  VariableName=sig_req_004_006  SaveFormat=Structure With Time
  ToWs_Req_Bus_Sig7 : ToWorkspace  VariableName=sig_req_004_007  SaveFormat=Structure With Time
  ToWs_Req_Bus_Sig8 : ToWorkspace  VariableName=sig_req_004_008  SaveFormat=Structure With Time
  ToWs_Req_Bus_Sig9 : ToWorkspace  VariableName=sig_req_004_009  SaveFormat=Structure With Time
  ToWs_Result_Bus_Sig1 : ToWorkspace  VariableName=sig_result_004_001  SaveFormat=Structure With Time
  ToWs_Result_Bus_Sig2 : ToWorkspace  VariableName=sig_result_004_002  SaveFormat=Structure With Time
  ToWs_Result_Bus_Sig3 : ToWorkspace  VariableName=sig_result_004_003  SaveFormat=Structure With Time
  specifyOutputs : Subsystem
  result : Outport
  wires:
  sig_Req_Bus/1 -> BS/1, specifyOutputs/1(sig_Req_Bus)
  BS/1 -> ToWs_Req_Bus_Sig1/1  "<testSig_T15_st>"
  BS/2 -> ToWs_Req_Bus_Sig2/1  "<testSig_CoEng_st>"
  BS/3 -> ToWs_Req_Bus_Sig3/1  "<testSig_Epm_nEng>"
  BS/4 -> ToWs_Req_Bus_Sig4/1  "<testSig_BattU_u>"
  BS/5 -> ToWs_Req_Bus_Sig5/1  "<testSig_CEngDsT_t>"
  BS/6 -> ToWs_Req_Bus_Sig6/1  "<testSig_FuelT_t>"
  BS/7 -> ToWs_Req_Bus_Sig7/1  "<testSig_Oil_tSwmp>"
  BS/8 -> ToWs_Req_Bus_Sig8/1  "<testSig_Air_tCACDs_mp>"
  BS/9 -> ToWs_Req_Bus_Sig9/1  "<testSig_Air_tAFS_mp>"
  BS/10 -> ToWs_Req_Bus_Sig10/1  "<testSig_EnvT_t>"
  BS/11 -> ToWs_Req_Bus_Sig11/1  "<testSig_Air_tIntkVUs>"
  BS/12 -> ToWs_Req_Bus_Sig12/1  "<testSig_DSM_bAirHtCEngDsT>"
  BS/13 -> ToWs_Req_Bus_Sig13/1  "<testSig_DSM_bAirHtFuelT>"
  BS/14 -> ToWs_Req_Bus_Sig14/1  "<testSig_DSM_bAirHtOilT>"
  BS/15 -> ToWs_Req_Bus_Sig15/1  "<testSig_DSM_bAirHtEnvT>"
  BS/16 -> ToWs_Req_Bus_Sig16/1  "<testSig_DSM_bAirHtCACDs>"
  BS/17 -> ToWs_Req_Bus_Sig17/1  "<testSig_DSM_bAirHtAFST>"
  BS/18 -> ToWs_Req_Bus_Sig18/1  "<testSig_DSM_bAirHtIntkVUsT>"
  BS/19 -> ToWs_Req_Bus_Sig19/1  "<testSig_AirHt_st>"
  BS/20 -> ToWs_Req_Bus_Sig20/1  "<testSig_IAirHt_st>"
  BS/21 -> ToWs_Req_Bus_Sig21/1  "<testSig_GlwLmp_st>"
  sig_Result_Bus/1 -> BS_Result/1, specifyOutputs/2(sig_Result_Bus)
  BS_Result/1 -> ToWs_Result_Bus_Sig1/1  "<AirHt_st>"
  BS_Result/2 -> ToWs_Result_Bus_Sig2/1  "<IAirHt_st>"
  BS_Result/3 -> ToWs_Result_Bus_Sig3/1  "<GlwLmp_st>"
  specifyOutputs/1(result) -> result/1

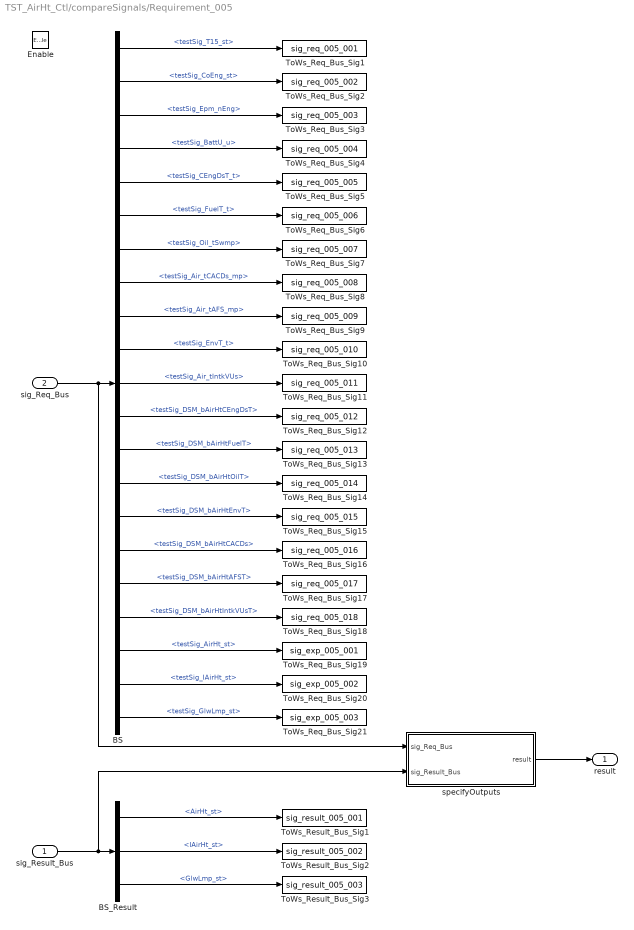
== system TST_AirHt_Ctl/compareSignals/Requirement_005 ==
  sig_Result_Bus : Inport
  sig_Req_Bus : Inport  Port=2
  Enable : EnablePort
  BS : BusSelector  OutputSignals=testSig_T15_st,testSig_CoEng_st,testSig_Epm_nEng,testSig_BattU_u,testSig_CEngDsT_t,testSig_FuelT_t,testSig_Oil_tSwmp,testSig_Air_tCACDs_mp,testSig_Air_tAFS_mp,testSig_EnvT_t,testSig_Air_tIntkVUs,testSig_DSM_bAirHtCEngDsT,testSig_DSM_bAirHtFuelT,testSig_DSM_bAirHtOilT,testSig_DSM_bAirHtEnvT,testSig_DSM_bAirHtCACDs,testSig_DSM_bAirHtAFST,testSig_DSM_bAirHtIntkVUsT,testSig_AirHt_st,testSig_IAirHt_st,testSig_GlwLmp_st
  BS_Result : BusSelector  OutputSignals=AirHt_st,IAirHt_st,GlwLmp_st
  ToWs_Req_Bus_Sig1 : ToWorkspace  VariableName=sig_req_005_001  SaveFormat=Structure With Time
  ToWs_Req_Bus_Sig10 : ToWorkspace  VariableName=sig_req_005_010  SaveFormat=Structure With Time
  ToWs_Req_Bus_Sig11 : ToWorkspace  VariableName=sig_req_005_011  SaveFormat=Structure With Time
  ToWs_Req_Bus_Sig12 : ToWorkspace  VariableName=sig_req_005_012  SaveFormat=Structure With Time
  ToWs_Req_Bus_Sig13 : ToWorkspace  VariableName=sig_req_005_013  SaveFormat=Structure With Time
  ToWs_Req_Bus_Sig14 : ToWorkspace  VariableName=sig_req_005_014  SaveFormat=Structure With Time
  ToWs_Req_Bus_Sig15 : ToWorkspace  VariableName=sig_req_005_015  SaveFormat=Structure With Time
  ToWs_Req_Bus_Sig16 : ToWorkspace  VariableName=sig_req_005_016  SaveFormat=Structure With Time
  ToWs_Req_Bus_Sig17 : ToWorkspace  VariableName=sig_req_005_017  SaveFormat=Structure With Time
  ToWs_Req_Bus_Sig18 : ToWorkspace  VariableName=sig_req_005_018  SaveFormat=Structure With Time
  ToWs_Req_Bus_Sig19 : ToWorkspace  VariableName=sig_exp_005_001  SaveFormat=Structure With Time
  ToWs_Req_Bus_Sig2 : ToWorkspace  VariableName=sig_req_005_002  SaveFormat=Structure With Time
  ToWs_Req_Bus_Sig20 : ToWorkspace  VariableName=sig_exp_005_002  SaveFormat=Structure With Time
  ToWs_Req_Bus_Sig21 : ToWorkspace  VariableName=sig_exp_005_003  SaveFormat=Structure With Time
  ToWs_Req_Bus_Sig3 : ToWorkspace  VariableName=sig_req_005_003  SaveFormat=Structure With Time
  ToWs_Req_Bus_Sig4 : ToWorkspace  VariableName=sig_req_005_004  SaveFormat=Structure With Time
  ToWs_Req_Bus_Sig5 : ToWorkspace  VariableName=sig_req_005_005  SaveFormat=Structure With Time
  ToWs_Req_Bus_Sig6 : ToWorkspace  VariableName=sig_req_005_006  SaveFormat=Structure With Time
  ToWs_Req_Bus_Sig7 : ToWorkspace  VariableName=sig_req_005_007  SaveFormat=Structure With Time
  ToWs_Req_Bus_Sig8 : ToWorkspace  VariableName=sig_req_005_008  SaveFormat=Structure With Time
  ToWs_Req_Bus_Sig9 : ToWorkspace  VariableName=sig_req_005_009  SaveFormat=Structure With Time
  ToWs_Result_Bus_Sig1 : ToWorkspace  VariableName=sig_result_005_001  SaveFormat=Structure With Time
  ToWs_Result_Bus_Sig2 : ToWorkspace  VariableName=sig_result_005_002  SaveFormat=Structure With Time
  ToWs_Result_Bus_Sig3 : ToWorkspace  VariableName=sig_result_005_003  SaveFormat=Structure With Time
  specifyOutputs : Subsystem
  result : Outport
  wires:
  sig_Req_Bus/1 -> BS/1, specifyOutputs/1(sig_Req_Bus)
  BS/1 -> ToWs_Req_Bus_Sig1/1  "<testSig_T15_st>"
  BS/2 -> ToWs_Req_Bus_Sig2/1  "<testSig_CoEng_st>"
  BS/3 -> ToWs_Req_Bus_Sig3/1  "<testSig_Epm_nEng>"
  BS/4 -> ToWs_Req_Bus_Sig4/1  "<testSig_BattU_u>"
  BS/5 -> ToWs_Req_Bus_Sig5/1  "<testSig_CEngDsT_t>"
  BS/6 -> ToWs_Req_Bus_Sig6/1  "<testSig_FuelT_t>"
  BS/7 -> ToWs_Req_Bus_Sig7/1  "<testSig_Oil_tSwmp>"
  BS/8 -> ToWs_Req_Bus_Sig8/1  "<testSig_Air_tCACDs_mp>"
  BS/9 -> ToWs_Req_Bus_Sig9/1  "<testSig_Air_tAFS_mp>"
  BS/10 -> ToWs_Req_Bus_Sig10/1  "<testSig_EnvT_t>"
  BS/11 -> ToWs_Req_Bus_Sig11/1  "<testSig_Air_tIntkVUs>"
  BS/12 -> ToWs_Req_Bus_Sig12/1  "<testSig_DSM_bAirHtCEngDsT>"
  BS/13 -> ToWs_Req_Bus_Sig13/1  "<testSig_DSM_bAirHtFuelT>"
  BS/14 -> ToWs_Req_Bus_Sig14/1  "<testSig_DSM_bAirHtOilT>"
  BS/15 -> ToWs_Req_Bus_Sig15/1  "<testSig_DSM_bAirHtEnvT>"
  BS/16 -> ToWs_Req_Bus_Sig16/1  "<testSig_DSM_bAirHtCACDs>"
  BS/17 -> ToWs_Req_Bus_Sig17/1  "<testSig_DSM_bAirHtAFST>"
  BS/18 -> ToWs_Req_Bus_Sig18/1  "<testSig_DSM_bAirHtIntkVUsT>"
  BS/19 -> ToWs_Req_Bus_Sig19/1  "<testSig_AirHt_st>"
  BS/20 -> ToWs_Req_Bus_Sig20/1  "<testSig_IAirHt_st>"
  BS/21 -> ToWs_Req_Bus_Sig21/1  "<testSig_GlwLmp_st>"
  sig_Result_Bus/1 -> BS_Result/1, specifyOutputs/2(sig_Result_Bus)
  BS_Result/1 -> ToWs_Result_Bus_Sig1/1  "<AirHt_st>"
  BS_Result/2 -> ToWs_Result_Bus_Sig2/1  "<IAirHt_st>"
  BS_Result/3 -> ToWs_Result_Bus_Sig3/1  "<GlwLmp_st>"
  specifyOutputs/1(result) -> result/1

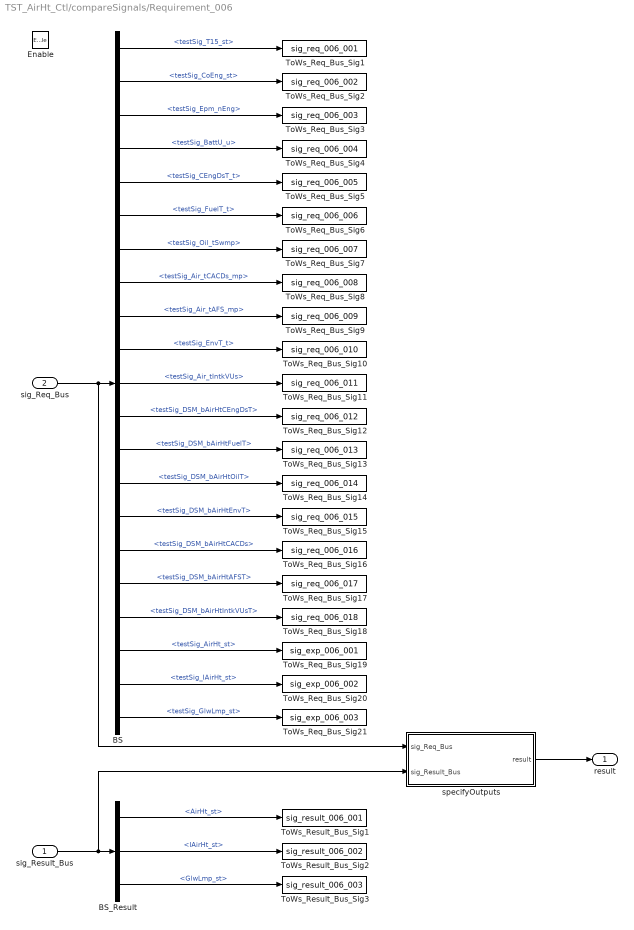
== system TST_AirHt_Ctl/compareSignals/Requirement_006 ==
  sig_Result_Bus : Inport
  sig_Req_Bus : Inport  Port=2
  Enable : EnablePort
  BS : BusSelector  OutputSignals=testSig_T15_st,testSig_CoEng_st,testSig_Epm_nEng,testSig_BattU_u,testSig_CEngDsT_t,testSig_FuelT_t,testSig_Oil_tSwmp,testSig_Air_tCACDs_mp,testSig_Air_tAFS_mp,testSig_EnvT_t,testSig_Air_tIntkVUs,testSig_DSM_bAirHtCEngDsT,testSig_DSM_bAirHtFuelT,testSig_DSM_bAirHtOilT,testSig_DSM_bAirHtEnvT,testSig_DSM_bAirHtCACDs,testSig_DSM_bAirHtAFST,testSig_DSM_bAirHtIntkVUsT,testSig_AirHt_st,testSig_IAirHt_st,testSig_GlwLmp_st
  BS_Result : BusSelector  OutputSignals=AirHt_st,IAirHt_st,GlwLmp_st
  ToWs_Req_Bus_Sig1 : ToWorkspace  VariableName=sig_req_006_001  SaveFormat=Structure With Time
  ToWs_Req_Bus_Sig10 : ToWorkspace  VariableName=sig_req_006_010  SaveFormat=Structure With Time
  ToWs_Req_Bus_Sig11 : ToWorkspace  VariableName=sig_req_006_011  SaveFormat=Structure With Time
  ToWs_Req_Bus_Sig12 : ToWorkspace  VariableName=sig_req_006_012  SaveFormat=Structure With Time
  ToWs_Req_Bus_Sig13 : ToWorkspace  VariableName=sig_req_006_013  SaveFormat=Structure With Time
  ToWs_Req_Bus_Sig14 : ToWorkspace  VariableName=sig_req_006_014  SaveFormat=Structure With Time
  ToWs_Req_Bus_Sig15 : ToWorkspace  VariableName=sig_req_006_015  SaveFormat=Structure With Time
  ToWs_Req_Bus_Sig16 : ToWorkspace  VariableName=sig_req_006_016  SaveFormat=Structure With Time
  ToWs_Req_Bus_Sig17 : ToWorkspace  VariableName=sig_req_006_017  SaveFormat=Structure With Time
  ToWs_Req_Bus_Sig18 : ToWorkspace  VariableName=sig_req_006_018  SaveFormat=Structure With Time
  ToWs_Req_Bus_Sig19 : ToWorkspace  VariableName=sig_exp_006_001  SaveFormat=Structure With Time
  ToWs_Req_Bus_Sig2 : ToWorkspace  VariableName=sig_req_006_002  SaveFormat=Structure With Time
  ToWs_Req_Bus_Sig20 : ToWorkspace  VariableName=sig_exp_006_002  SaveFormat=Structure With Time
  ToWs_Req_Bus_Sig21 : ToWorkspace  VariableName=sig_exp_006_003  SaveFormat=Structure With Time
  ToWs_Req_Bus_Sig3 : ToWorkspace  VariableName=sig_req_006_003  SaveFormat=Structure With Time
  ToWs_Req_Bus_Sig4 : ToWorkspace  VariableName=sig_req_006_004  SaveFormat=Structure With Time
  ToWs_Req_Bus_Sig5 : ToWorkspace  VariableName=sig_req_006_005  SaveFormat=Structure With Time
  ToWs_Req_Bus_Sig6 : ToWorkspace  VariableName=sig_req_006_006  SaveFormat=Structure With Time
  ToWs_Req_Bus_Sig7 : ToWorkspace  VariableName=sig_req_006_007  SaveFormat=Structure With Time
  ToWs_Req_Bus_Sig8 : ToWorkspace  VariableName=sig_req_006_008  SaveFormat=Structure With Time
  ToWs_Req_Bus_Sig9 : ToWorkspace  VariableName=sig_req_006_009  SaveFormat=Structure With Time
  ToWs_Result_Bus_Sig1 : ToWorkspace  VariableName=sig_result_006_001  SaveFormat=Structure With Time
  ToWs_Result_Bus_Sig2 : ToWorkspace  VariableName=sig_result_006_002  SaveFormat=Structure With Time
  ToWs_Result_Bus_Sig3 : ToWorkspace  VariableName=sig_result_006_003  SaveFormat=Structure With Time
  specifyOutputs : Subsystem
  result : Outport
  wires:
  sig_Req_Bus/1 -> BS/1, specifyOutputs/1(sig_Req_Bus)
  BS/1 -> ToWs_Req_Bus_Sig1/1  "<testSig_T15_st>"
  BS/2 -> ToWs_Req_Bus_Sig2/1  "<testSig_CoEng_st>"
  BS/3 -> ToWs_Req_Bus_Sig3/1  "<testSig_Epm_nEng>"
  BS/4 -> ToWs_Req_Bus_Sig4/1  "<testSig_BattU_u>"
  BS/5 -> ToWs_Req_Bus_Sig5/1  "<testSig_CEngDsT_t>"
  BS/6 -> ToWs_Req_Bus_Sig6/1  "<testSig_FuelT_t>"
  BS/7 -> ToWs_Req_Bus_Sig7/1  "<testSig_Oil_tSwmp>"
  BS/8 -> ToWs_Req_Bus_Sig8/1  "<testSig_Air_tCACDs_mp>"
  BS/9 -> ToWs_Req_Bus_Sig9/1  "<testSig_Air_tAFS_mp>"
  BS/10 -> ToWs_Req_Bus_Sig10/1  "<testSig_EnvT_t>"
  BS/11 -> ToWs_Req_Bus_Sig11/1  "<testSig_Air_tIntkVUs>"
  BS/12 -> ToWs_Req_Bus_Sig12/1  "<testSig_DSM_bAirHtCEngDsT>"
  BS/13 -> ToWs_Req_Bus_Sig13/1  "<testSig_DSM_bAirHtFuelT>"
  BS/14 -> ToWs_Req_Bus_Sig14/1  "<testSig_DSM_bAirHtOilT>"
  BS/15 -> ToWs_Req_Bus_Sig15/1  "<testSig_DSM_bAirHtEnvT>"
  BS/16 -> ToWs_Req_Bus_Sig16/1  "<testSig_DSM_bAirHtCACDs>"
  BS/17 -> ToWs_Req_Bus_Sig17/1  "<testSig_DSM_bAirHtAFST>"
  BS/18 -> ToWs_Req_Bus_Sig18/1  "<testSig_DSM_bAirHtIntkVUsT>"
  BS/19 -> ToWs_Req_Bus_Sig19/1  "<testSig_AirHt_st>"
  BS/20 -> ToWs_Req_Bus_Sig20/1  "<testSig_IAirHt_st>"
  BS/21 -> ToWs_Req_Bus_Sig21/1  "<testSig_GlwLmp_st>"
  sig_Result_Bus/1 -> BS_Result/1, specifyOutputs/2(sig_Result_Bus)
  BS_Result/1 -> ToWs_Result_Bus_Sig1/1  "<AirHt_st>"
  BS_Result/2 -> ToWs_Result_Bus_Sig2/1  "<IAirHt_st>"
  BS_Result/3 -> ToWs_Result_Bus_Sig3/1  "<GlwLmp_st>"
  specifyOutputs/1(result) -> result/1

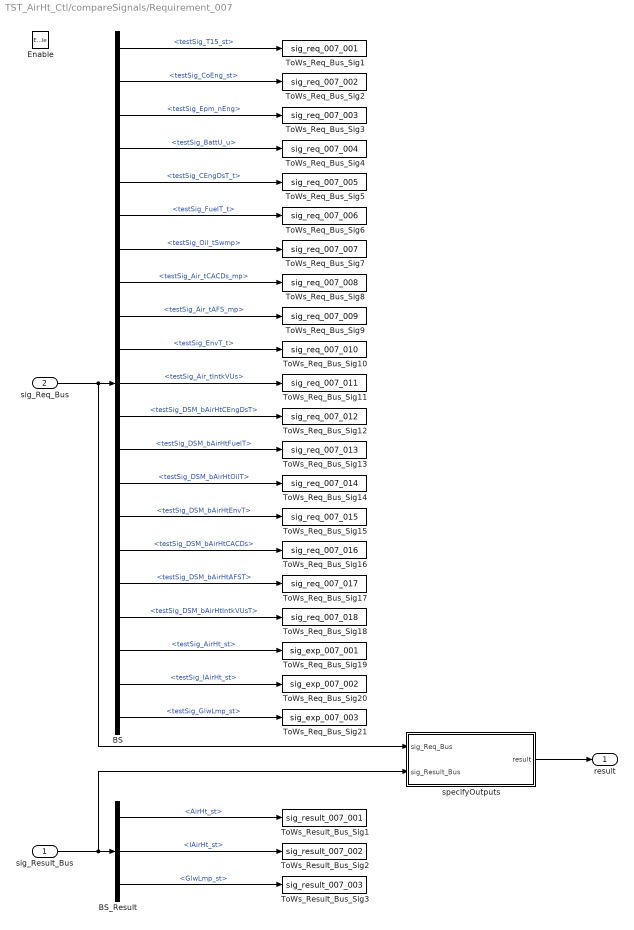
== system TST_AirHt_Ctl/compareSignals/Requirement_007 ==
  sig_Result_Bus : Inport
  sig_Req_Bus : Inport  Port=2
  Enable : EnablePort
  BS : BusSelector  OutputSignals=testSig_T15_st,testSig_CoEng_st,testSig_Epm_nEng,testSig_BattU_u,testSig_CEngDsT_t,testSig_FuelT_t,testSig_Oil_tSwmp,testSig_Air_tCACDs_mp,testSig_Air_tAFS_mp,testSig_EnvT_t,testSig_Air_tIntkVUs,testSig_DSM_bAirHtCEngDsT,testSig_DSM_bAirHtFuelT,testSig_DSM_bAirHtOilT,testSig_DSM_bAirHtEnvT,testSig_DSM_bAirHtCACDs,testSig_DSM_bAirHtAFST,testSig_DSM_bAirHtIntkVUsT,testSig_AirHt_st,testSig_IAirHt_st,testSig_GlwLmp_st
  BS_Result : BusSelector  OutputSignals=AirHt_st,IAirHt_st,GlwLmp_st
  ToWs_Req_Bus_Sig1 : ToWorkspace  VariableName=sig_req_007_001  SaveFormat=Structure With Time
  ToWs_Req_Bus_Sig10 : ToWorkspace  VariableName=sig_req_007_010  SaveFormat=Structure With Time
  ToWs_Req_Bus_Sig11 : ToWorkspace  VariableName=sig_req_007_011  SaveFormat=Structure With Time
  ToWs_Req_Bus_Sig12 : ToWorkspace  VariableName=sig_req_007_012  SaveFormat=Structure With Time
  ToWs_Req_Bus_Sig13 : ToWorkspace  VariableName=sig_req_007_013  SaveFormat=Structure With Time
  ToWs_Req_Bus_Sig14 : ToWorkspace  VariableName=sig_req_007_014  SaveFormat=Structure With Time
  ToWs_Req_Bus_Sig15 : ToWorkspace  VariableName=sig_req_007_015  SaveFormat=Structure With Time
  ToWs_Req_Bus_Sig16 : ToWorkspace  VariableName=sig_req_007_016  SaveFormat=Structure With Time
  ToWs_Req_Bus_Sig17 : ToWorkspace  VariableName=sig_req_007_017  SaveFormat=Structure With Time
  ToWs_Req_Bus_Sig18 : ToWorkspace  VariableName=sig_req_007_018  SaveFormat=Structure With Time
  ToWs_Req_Bus_Sig19 : ToWorkspace  VariableName=sig_exp_007_001  SaveFormat=Structure With Time
  ToWs_Req_Bus_Sig2 : ToWorkspace  VariableName=sig_req_007_002  SaveFormat=Structure With Time
  ToWs_Req_Bus_Sig20 : ToWorkspace  VariableName=sig_exp_007_002  SaveFormat=Structure With Time
  ToWs_Req_Bus_Sig21 : ToWorkspace  VariableName=sig_exp_007_003  SaveFormat=Structure With Time
  ToWs_Req_Bus_Sig3 : ToWorkspace  VariableName=sig_req_007_003  SaveFormat=Structure With Time
  ToWs_Req_Bus_Sig4 : ToWorkspace  VariableName=sig_req_007_004  SaveFormat=Structure With Time
  ToWs_Req_Bus_Sig5 : ToWorkspace  VariableName=sig_req_007_005  SaveFormat=Structure With Time
  ToWs_Req_Bus_Sig6 : ToWorkspace  VariableName=sig_req_007_006  SaveFormat=Structure With Time
  ToWs_Req_Bus_Sig7 : ToWorkspace  VariableName=sig_req_007_007  SaveFormat=Structure With Time
  ToWs_Req_Bus_Sig8 : ToWorkspace  VariableName=sig_req_007_008  SaveFormat=Structure With Time
  ToWs_Req_Bus_Sig9 : ToWorkspace  VariableName=sig_req_007_009  SaveFormat=Structure With Time
  ToWs_Result_Bus_Sig1 : ToWorkspace  VariableName=sig_result_007_001  SaveFormat=Structure With Time
  ToWs_Result_Bus_Sig2 : ToWorkspace  VariableName=sig_result_007_002  SaveFormat=Structure With Time
  ToWs_Result_Bus_Sig3 : ToWorkspace  VariableName=sig_result_007_003  SaveFormat=Structure With Time
  specifyOutputs : Subsystem
  result : Outport
  wires:
  sig_Req_Bus/1 -> BS/1, specifyOutputs/1(sig_Req_Bus)
  BS/1 -> ToWs_Req_Bus_Sig1/1  "<testSig_T15_st>"
  BS/2 -> ToWs_Req_Bus_Sig2/1  "<testSig_CoEng_st>"
  BS/3 -> ToWs_Req_Bus_Sig3/1  "<testSig_Epm_nEng>"
  BS/4 -> ToWs_Req_Bus_Sig4/1  "<testSig_BattU_u>"
  BS/5 -> ToWs_Req_Bus_Sig5/1  "<testSig_CEngDsT_t>"
  BS/6 -> ToWs_Req_Bus_Sig6/1  "<testSig_FuelT_t>"
  BS/7 -> ToWs_Req_Bus_Sig7/1  "<testSig_Oil_tSwmp>"
  BS/8 -> ToWs_Req_Bus_Sig8/1  "<testSig_Air_tCACDs_mp>"
  BS/9 -> ToWs_Req_Bus_Sig9/1  "<testSig_Air_tAFS_mp>"
  BS/10 -> ToWs_Req_Bus_Sig10/1  "<testSig_EnvT_t>"
  BS/11 -> ToWs_Req_Bus_Sig11/1  "<testSig_Air_tIntkVUs>"
  BS/12 -> ToWs_Req_Bus_Sig12/1  "<testSig_DSM_bAirHtCEngDsT>"
  BS/13 -> ToWs_Req_Bus_Sig13/1  "<testSig_DSM_bAirHtFuelT>"
  BS/14 -> ToWs_Req_Bus_Sig14/1  "<testSig_DSM_bAirHtOilT>"
  BS/15 -> ToWs_Req_Bus_Sig15/1  "<testSig_DSM_bAirHtEnvT>"
  BS/16 -> ToWs_Req_Bus_Sig16/1  "<testSig_DSM_bAirHtCACDs>"
  BS/17 -> ToWs_Req_Bus_Sig17/1  "<testSig_DSM_bAirHtAFST>"
  BS/18 -> ToWs_Req_Bus_Sig18/1  "<testSig_DSM_bAirHtIntkVUsT>"
  BS/19 -> ToWs_Req_Bus_Sig19/1  "<testSig_AirHt_st>"
  BS/20 -> ToWs_Req_Bus_Sig20/1  "<testSig_IAirHt_st>"
  BS/21 -> ToWs_Req_Bus_Sig21/1  "<testSig_GlwLmp_st>"
  sig_Result_Bus/1 -> BS_Result/1, specifyOutputs/2(sig_Result_Bus)
  BS_Result/1 -> ToWs_Result_Bus_Sig1/1  "<AirHt_st>"
  BS_Result/2 -> ToWs_Result_Bus_Sig2/1  "<IAirHt_st>"
  BS_Result/3 -> ToWs_Result_Bus_Sig3/1  "<GlwLmp_st>"
  specifyOutputs/1(result) -> result/1
